simulink model "comparacao"  (R2019a)
settings: Solver=VariableStepAuto  StartTime=0.0  StopTime=1500  RelTol=1e-3
settings Model: Creator=josefernandorosaribeiro  LastModifiedBy=josefernandorosaribeiro

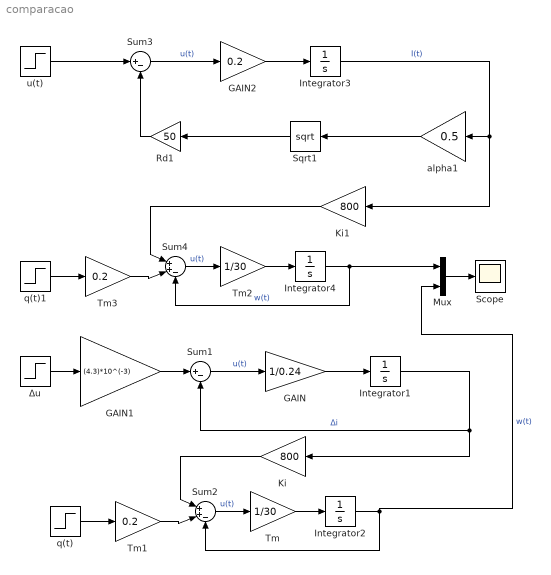
== system comparacao ==
  GAIN : Gain  Gain=1/0.24
  GAIN1 : Gain  Gain=(4.3)*10^(-3)
  GAIN2 : Gain  Gain=0.2
  Integrator{1..4} (4 alike) : Integrator  InitialCondition=0.0072
  Ki : Gain  Gain=800
  Ki1 : Gain  Gain=800
  Mux : Mux  Inputs=2
  Rd1 : Gain  Gain=50
  Scope : Scope
  Sqrt1 : Sqrt  SaturateOnIntegerOverflow=on
  Sum1 : Sum  Inputs=|+-
  Sum2 : Sum  Inputs=|++-
  Sum3 : Sum  Inputs=|+-
  Sum4 : Sum  Inputs=|++-
  Tm : Gain  Gain=1/30
  Tm1 : Gain  Gain=0.2
  Tm2 : Gain  Gain=1/30
  Tm3 : Gain  Gain=0.2
  alpha1 : Gain  Gain=0.5
  q(t) : Step  Before=5  After=5  SampleTime=0
  q(t)1 : Step  Before=5  After=5  SampleTime=0
  u(t) : Step  Before=1  After=5  SampleTime=0
  Δu : Step  Before=1  After=5  SampleTime=0
  wires:
  Δu/1 -> GAIN1/1
  Sum1/1 -> GAIN/1  "u(t)"
  GAIN/1 -> Integrator1/1
  Integrator1/1 -> Sum1/2, Ki/1  "Δi"
  Integrator2/1 -> Mux/2, Sum2/3  "w(t)"
  Sum2/1 -> Tm/1  "u(t)"
  Tm/1 -> Integrator2/1
  Ki/1 -> Sum2/1
  q(t)/1 -> Tm1/1
  Tm1/1 -> Sum2/2
  GAIN1/1 -> Sum1/1
  GAIN2/1 -> Integrator3/1
  Sum4/1 -> Tm2/1  "u(t)"
  Rd1/1 -> Sum3/2
  Sqrt1/1 -> Rd1/1
  Tm2/1 -> Integrator4/1
  q(t)1/1 -> Tm3/1
  alpha1/1 -> Sqrt1/1
  Integrator3/1 -> Ki1/1, alpha1/1  "I(t)"
  Ki1/1 -> Sum4/1
  Tm3/1 -> Sum4/2
  Integrator4/1 -> Mux/1, Sum4/3  "w(t)"
  Sum3/1 -> GAIN2/1  "u(t)"
  u(t)/1 -> Sum3/1
  Mux/1 -> Scope/1
